simulink model "as2"  (Simulink 8.4)
settings: Solver=ode45  StartTime=0.0  StopTime=50  RelTol=1e-7
settings Model: Creator=Administrator  LastModifiedBy=zhouy
settings DataIOCC: SignalLoggingSaveFormat=Dataset
settings OptimizationCC: ExpressionDepthLimit=128
settings DebuggingCC: UnderspecifiedInitializationDetection=Simplified  MergeDetectMultiDrivingBlocksExec=error  FcnCallInpInsideContextMsg=EnableAllAsError  StateNameClashWarn=none
settings GRTTargetCC: CombineOutputUpdateFcns=on  GRTInterface=off

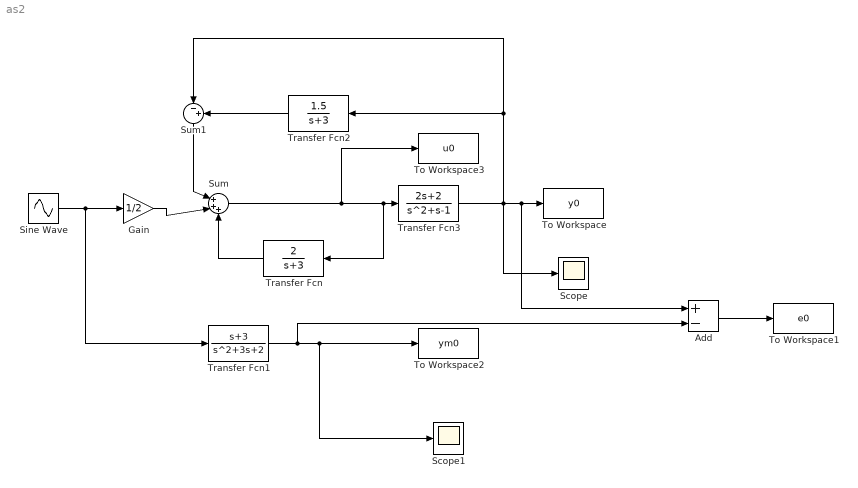
== system as2 ==
  Add : Sum  Inputs=+-
  Gain : Gain  Gain=1/2
  Scope : Scope
  Scope1 : Scope
  Sine Wave : Sin  SampleTime=0
  Sum : Sum  Inputs=|+++
  Sum1 : Sum  Inputs=|-+
  To Workspace : ToWorkspace  VariableName=y0  SaveFormat=Timeseries  SampleTime=-1
  To Workspace1 : ToWorkspace  VariableName=e0  SaveFormat=Timeseries  SampleTime=-1
  To Workspace2 : ToWorkspace  VariableName=ym0  SaveFormat=Timeseries  SampleTime=-1
  To Workspace3 : ToWorkspace  VariableName=u0  SaveFormat=Timeseries  SampleTime=-1
  Transfer Fcn : TransferFcn  Numerator=[2]  Denominator=[1 3]
  Transfer Fcn1 : TransferFcn  Numerator=[1 3]  Denominator=[1 3 2]
  Transfer Fcn2 : TransferFcn  Numerator=[1.5]  Denominator=[1 3]
  Transfer Fcn3 : TransferFcn  Numerator=[2 2]  Denominator=[1 1 -1]
  wires:
  Sum/1 -> To Workspace3/1, Transfer Fcn/1, Transfer Fcn3/1
  Transfer Fcn3/1 -> Add/1, To Workspace/1, Scope/1, Transfer Fcn2/1, Sum1/1
  Sine Wave/1 -> Transfer Fcn1/1, Gain/1
  Gain/1 -> Sum/2
  Transfer Fcn1/1 -> Add/2, Scope1/1, To Workspace2/1
  Transfer Fcn/1 -> Sum/3
  Transfer Fcn2/1 -> Sum1/2
  Sum1/1 -> Sum/1
  Add/1 -> To Workspace1/1
